simulink model "cpe348_project1_simulink"  (R2024a)
settings: Solver=VariableStepAuto  StartTime=0.0  StopTime=20.0  RelTol=1e-3
libraries: commutil2 x2
settings Model: Creator=eshore  LastModifiedBy=eshore

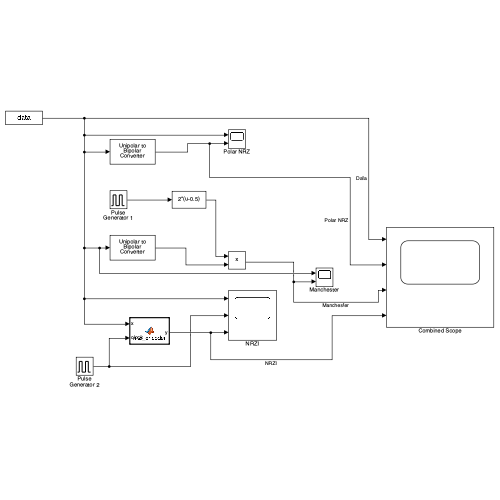
[thumbnail: Simulink's stored preview of the top-level diagram]
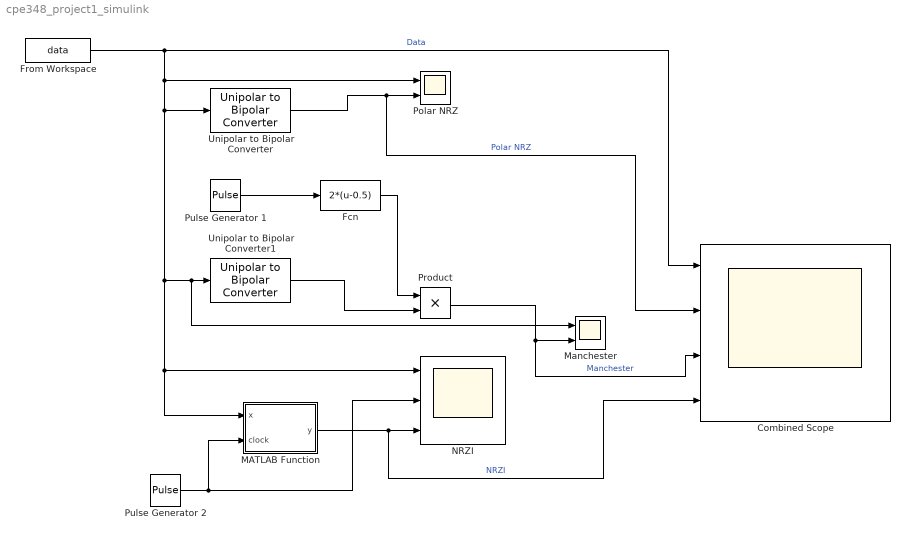
== system cpe348_project1_simulink ==
  Combined Scope : Scope  NumInputPorts=4
  Fcn : Fcn  Expr=2*(u-0.5)
  From Workspace : FromWorkspace  VariableName=data  SampleTime=1  OutputAfterFinalValue=Setting to zero
  MATLAB Function : MATLAB Function  TreatAsAtomicUnit=on
  Manchester : Scope  NumInputPorts=2
  NRZI : Scope  NumInputPorts=3
  Polar NRZ : Scope  NumInputPorts=2
  Product : Product
  Pulse Generator 1 : DiscretePulseGenerator  PulseType=Time based  Period=1  PulseWidth=50
  Pulse Generator 2 : DiscretePulseGenerator  PulseType=Time based  Period=1  PulseWidth=50  PhaseDelay=0.5
  Unipolar to Bipolar Converter : commutil2/Unipolar to Bipolar Converter  M=2  polarity=Positive  dataType=Inherit via internal rule
  Unipolar to Bipolar Converter1 : commutil2/Unipolar to Bipolar Converter  M=2  polarity=Positive  dataType=Inherit via internal rule
  wires:
  Pulse Generator 2/1 -> MATLAB Function/2(clock), NRZI/2
  From Workspace/1 -> Combined Scope/1, Polar NRZ/1, MATLAB Function/1(x), NRZI/1, Manchester/1, Unipolar to Bipolar Converter1/1, Unipolar to Bipolar Converter/1  "Data"
  Pulse Generator 1/1 -> Fcn/1
  Unipolar to Bipolar Converter1/1 -> Product/2
  Fcn/1 -> Product/1
  Product/1 -> Combined Scope/3, Manchester/2  "Manchester"
  Unipolar to Bipolar Converter/1 -> Combined Scope/2, Polar NRZ/2  "Polar NRZ"
  MATLAB Function/1(y) -> Combined Scope/4, NRZI/3  "NRZI"

== matlab function cpe348_project1_simulink/MATLAB Function ==
  data: x input; y output; clock input
function y  = nrzi_encoder(x, clock)
    % maintain values from previous function calls
    persistent last_y;
    persistent last_clk;
    % set initial value for NRZI output
    if (isempty(last_y))
        last_y = -1;
    end
    % set initial value for clk
    if (isempty(last_clk))
        last_clk = 0;
    end
    % transition y when x is 1 and rising edge of clock, otherwise unchanged
    if (x == 1 && (last_clk == 0 && clock == 1))
        y = -last_y;
    else
        y = last_y;
    end
    % set new values for future reference
    last_y = y;
    last_clk = clock;
end
